simulink model "Simulaciones_punto_7"  (R2017a)
settings: Solver=VariableStepAuto  StartTime=0.0  StopTime=10  RelTol=1e-3
settings Model: Creator=franj  LastModifiedBy=franj

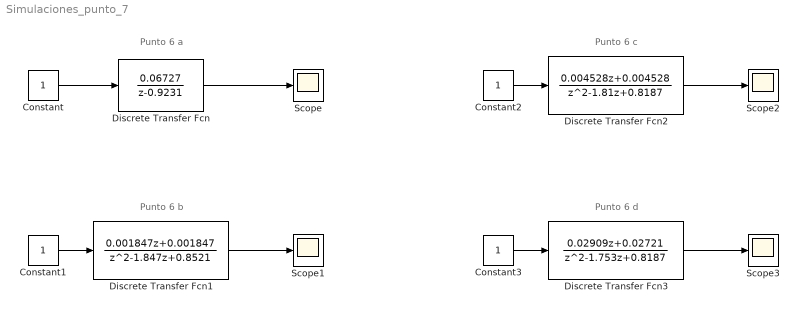
== system Simulaciones_punto_7 ==
  note: Punto 6 a
  note: Punto 6 b
  note: Punto 6 c
  note: Punto 6 d
  Constant{,1..3} (4 alike) : Constant
  Discrete Transfer Fcn : DiscreteTransferFcn  Numerator=[0.06727]  Denominator=[1 -0.9231]
  Discrete Transfer Fcn1 : DiscreteTransferFcn  Numerator=[0.001847 0.001847]  Denominator=[1 -1.847 0.8521]
  Discrete Transfer Fcn2 : DiscreteTransferFcn  Numerator=[0.004528 0.004528]  Denominator=[1 -1.81 0.8187]
  Discrete Transfer Fcn3 : DiscreteTransferFcn  Numerator=[0.02909 0.02721]  Denominator=[1 -1.753 0.8187]
  Scope{,1..3} (4 alike) : Scope
  wires:
  Constant/1 -> Discrete Transfer Fcn/1
  Discrete Transfer Fcn/1 -> Scope/1
  Constant1/1 -> Discrete Transfer Fcn1/1
  Discrete Transfer Fcn1/1 -> Scope1/1
  Constant2/1 -> Discrete Transfer Fcn2/1
  Discrete Transfer Fcn2/1 -> Scope2/1
  Discrete Transfer Fcn3/1 -> Scope3/1
  Constant3/1 -> Discrete Transfer Fcn3/1
